simulink model "TD3"  (R2024b)
settings: Solver=VariableStepAuto  StartTime=0.0  StopTime=10.0  RelTol=1e-3
values from neighbouring files (symbols this model uses):
  L = 1.6e-3    (= 0.0016)    [TD2_config.m]    (also in TD3_config.m)
  R = 0.13    [TD2_config.m]    (also in TD3_config.m)
settings Model: Creator=E306_PC2  LastModifiedBy=E306_PC2

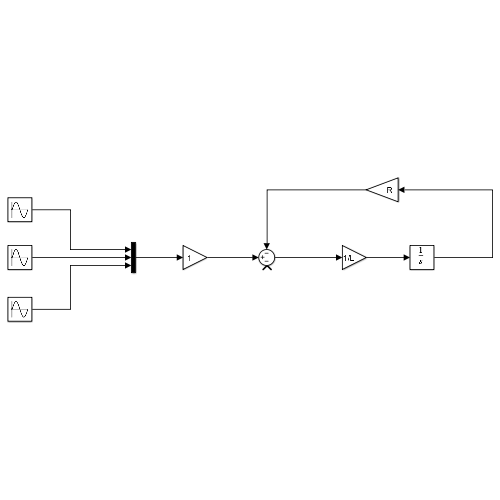
[thumbnail: Simulink's stored preview of the top-level diagram]
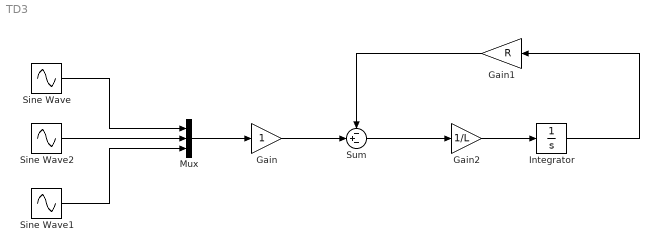
== system TD3 ==
  Gain : Gain
  Gain1 : Gain  Gain=R
  Gain2 : Gain  Gain=1/L
  Integrator : Integrator
  Mux : Mux  Inputs=3
  Sine Wave : Sin  SampleTime=0
  Sine Wave1 : Sin  SampleTime=0
  Sine Wave2 : Sin  SampleTime=0
  Sum : Sum  Inputs=-+-
  wires:
  Sine Wave/1 -> Mux/1
  Sine Wave2/1 -> Mux/2
  Sine Wave1/1 -> Mux/3
  Mux/1 -> Gain/1
  Gain/1 -> Sum/2
  Sum/1 -> Gain2/1
  Integrator/1 -> Gain1/1
  Gain1/1 -> Sum/1
  Gain2/1 -> Integrator/1
